simulink model "ICW_a1"  (Simulink 8.7)
settings: Solver=ode1  SolverMode=SingleTasking  StartTime=0.0  StopTime=500  FixedStep=0.001  RelTol=1e-3
(part 4 of 6)

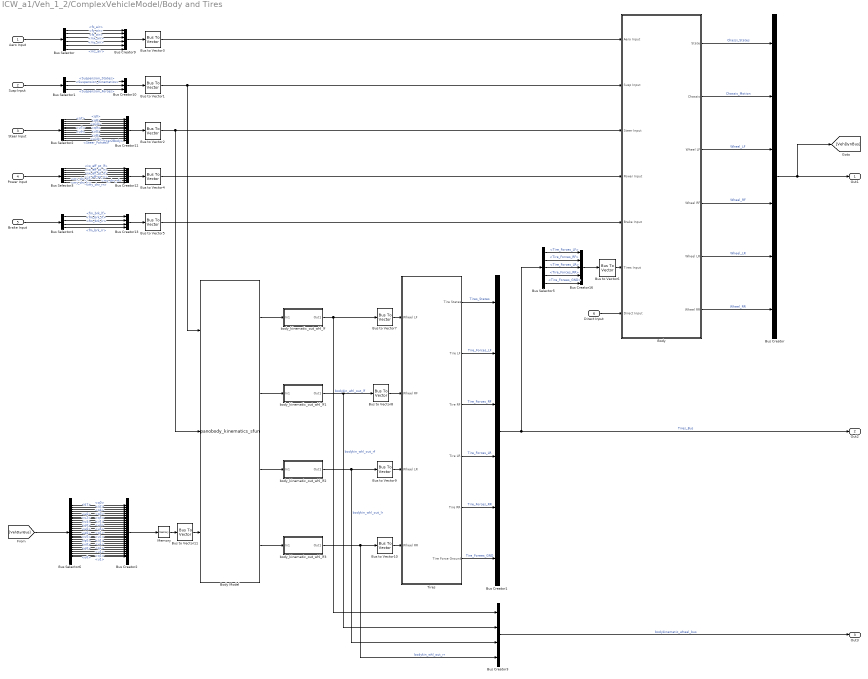
== system ICW_a1/Veh_1_2/ComplexVehicleModel/Body and Tires ==
  Aero Input : Inport
  Susp Input : Inport  Port=2
  Steer Input : Inport  Port=3
  Power Input : Inport  Port=4
  Brake Input : Inport  Port=5
  Direct Input : Inport  Port=6
  Body : Subsystem
  Body Model : S-Function  FunctionName=panobody_kinematics_sfun  Parameters='d84d7fde-53e6-4f2b-9c8e-847f55afb80f'  SFunctionDeploymentMode=off  EnableBusSupport=off
  Bus Creator : BusCreator  Inputs=6
  Bus Creator1 : BusCreator  Inputs=6
  Bus Creator10 : BusCreator  Inputs=3
  Bus Creator11 : BusCreator  Inputs=12
  Bus Creator12 : BusCreator  Inputs=8
  Bus Creator13 : BusCreator  Inputs=4
  Bus Creator16 : BusCreator  Inputs=5
  Bus Creator2 : BusCreator  Inputs=28
  Bus Creator3 : BusCreator  Inputs=4
  Bus Creator9 : BusCreator  Inputs=6
  Bus Selector : BusSelector  OutputSignals=Aerodynamics_Output.fx_air,Aerodynamics_Output.fy_air,Aerodynamics_Output.fz_air,Aerodynamics_Output.mx_air,Aerodynamics_Output.my_air,Aerodynamics_Output.mz_air
  Bus Selector1 : BusSelector  OutputSignals=Suspension_States,Suspension_Kinematics,Suspension_Forces
  Bus Selector2 : BusSelector  OutputSignals=Steer_States.q0,Steer_States.q7,Steer_States.q8,Steer_States.q9,Steer_States.q10,Steer_States.u0,Steer_States.u7,Steer_States.u8,Steer_States.u9,Steer_States.u10,Steer2Body,Steer_Forces
  Bus Selector3 : BusSelector  OutputSignals=Powertrain_Output.iw_eff_pt_lf,Powertrain_Output.iw_eff_pt_rf,Powertrain_Output.iw_eff_pt_lr,Powertrain_Output.iw_eff_pt_rr,Powertrain_Output.my_drv_lf,Powertrain_Output.my_drv_rf,Powertrain_Output.my_drv_lr,Powertrain_Output.my_drv_rr
  Bus Selector4 : BusSelector  OutputSignals=Brake_Output.fm_brk_lf,Brake_Output.fm_brk_rf,Brake_Output.fm_brk_lr,Brake_Output.fm_brk_rr
  Bus Selector5 : BusSelector  OutputSignals=Tire_Forces_LF,Tire_Forces_RF,Tire_Forces_LR,Tire_Forces_RR,Tire_Forees_GND
  Bus Selector6 : BusSelector  OutputSignals=Chassi_States.q0,Chassi_States.q1,Chassi_States.q2,Chassi_States.q3,Chassi_States.q4,Chassi_States.q5,Chassi_States.u0,Chassi_States.u1,Chassi_States.u2,Chassi_States.u3,Chassi_States.u4,Chassi_States.u5,Wheel_LF.q0,Wheel_LF.q1,Wheel_LF.u0,Wheel_LF.u1,Wheel_RF.q0,Wheel_RF.q1,Wheel_RF.u0,Wheel_RF.u1,Wheel_LR.q0,Wheel_LR.q1,Wheel_LR.u0,Wheel_LR.u1,Wheel_RR.q0,Wheel_RR.q1,Wheel_RR.u0,Wheel_RR.u1
  Bus to Vector{1..11} (11 alike) : BusToVector
  Memory : Memory
  Tires : Subsystem
  body_kinematic_out_whl_lf : Subsystem
  body_kinematic_out_whl_lf1 : Subsystem
  body_kinematic_out_whl_lf2 : Subsystem
  body_kinematic_out_whl_lf3 : Subsystem
  Out1 : Outport
  Out2 : Outport  Port=2
  Out3 : Outport  Port=3
  wires:
  Bus Selector5/5 -> Bus Creator16/5  "<Tire_Forees_GND>"
  Tires/6(Tire Force Ground) -> Bus Creator1/6  "Tire_Forees_GND"
  Aero Input/1 -> Bus Selector/1
  Susp Input/1 -> Bus Selector1/1
  Body/1(State) -> Bus Creator/1  "Chassi_States"
  Body/2(Chassis) -> Bus Creator/2  "Chassis_Motion"
  Body/3(Wheel LF) -> Bus Creator/3  "Wheel_LF"
  Body/4(Wheel RF) -> Bus Creator/4  "Wheel_RF"
  Body/5(Wheel LR) -> Bus Creator/5  "Wheel_LR"
  Body/6(Wheel RR) -> Bus Creator/6  "Wheel_RR"
  Bus Selector/1 -> Bus Creator9/1  "<fx_air>"
  Bus Selector/2 -> Bus Creator9/2  "<fy_air>"
  Bus Selector/3 -> Bus Creator9/3  "<fz_air>"
  Bus Selector/4 -> Bus Creator9/4  "<mx_air>"
  Bus Selector/5 -> Bus Creator9/5  "<my_air>"
  Bus Selector/6 -> Bus Creator9/6  "<mz_air>"
  Bus Selector1/1 -> Bus Creator10/1  "<Suspension_States>"
  Bus Selector1/2 -> Bus Creator10/2  "<Suspension_Kinematics>"
  Bus Selector3/1 -> Bus Creator12/1  "<iw_eff_pt_lf>"
  Bus Selector3/2 -> Bus Creator12/2  "<iw_eff_pt_rf>"
  Bus Selector3/3 -> Bus Creator12/3  "<iw_eff_pt_lr>"
  Bus Selector3/4 -> Bus Creator12/4  "<iw_eff_pt_rr>"
  Bus Selector4/1 -> Bus Creator13/1  "<fm_brk_lf>"
  Bus Selector4/2 -> Bus Creator13/2  "<fm_brk_rf>"
  Bus Selector4/3 -> Bus Creator13/3  "<fm_brk_lr>"
  Bus Selector4/4 -> Bus Creator13/4  "<fm_brk_rr>"
  Bus Selector5/1 -> Bus Creator16/1  "<Tire_Forces_LF>"
  Bus Selector5/2 -> Bus Creator16/2  "<Tire_Forces_RF>"
  Bus Selector5/3 -> Bus Creator16/3  "<Tire_Forces_LR>"
  Bus Selector5/4 -> Bus Creator16/4  "<Tire_Forces_RR>"
  Bus Creator16/1 -> Bus to Vector6/1
  Bus Selector2/1 -> Bus Creator11/1  "<q0>"
  Bus Selector2/2 -> Bus Creator11/2  "<q7>"
  Bus Selector2/3 -> Bus Creator11/3  "<q8>"
  Bus Selector2/4 -> Bus Creator11/4  "<q9>"
  Bus Selector2/5 -> Bus Creator11/5  "<q10>"
  Bus Selector2/6 -> Bus Creator11/6  "<u0>"
  Bus Selector2/7 -> Bus Creator11/7  "<u7>"
  Bus Selector2/8 -> Bus Creator11/8  "<u8>"
  Bus Selector2/9 -> Bus Creator11/9  "<u9>"
  Bus Selector2/10 -> Bus Creator11/10  "<u10>"
  Bus Selector2/11 -> Bus Creator11/11  "<Steer2Body>"
  Bus Selector2/12 -> Bus Creator11/12  "<Steer_Forces>"
  Bus Creator/1 -> Out1/1, [VehDynBus]
  Tires/1(Tire States) -> Bus Creator1/1  "Tires_States"
  Tires/2(Tire LF) -> Bus Creator1/2  "Tire_Forces_LF"
  Tires/3(Tire RF) -> Bus Creator1/3  "Tire_Forces_RF"
  Tires/4(Tire LR) -> Bus Creator1/4  "Tire_Forces_LR"
  Tires/5(Tire RR) -> Bus Creator1/5  "Tire_Forces_RR"
  Bus Creator1/1 -> Bus Selector5/1, Out2/1  "Tires_Bus"
  Power Input/1 -> Bus Selector3/1
  Direct Input/1 -> Body/7(Direct Input)
  Brake Input/1 -> Bus Selector4/1
  Body Model/1 -> body_kinematic_out_whl_lf/1(In1)
  Body Model/2 -> body_kinematic_out_whl_lf1/1(In1)
  Body Model/3 -> body_kinematic_out_whl_lf2/1(In1)
  Body Model/4 -> body_kinematic_out_whl_lf3/1(In1)
  Steer Input/1 -> Bus Selector2/1
  Bus Selector1/3 -> Bus Creator10/3  "<Suspension_Forces>"
  Bus Selector3/5 -> Bus Creator12/5  "<my_drv_lf>"
  Bus Selector3/6 -> Bus Creator12/6  "<my_drv_rf>"
  Bus Selector3/7 -> Bus Creator12/7  "<my_drv_lr>"
  Bus Selector3/8 -> Bus Creator12/8  "<my_drv_rr>"
  Bus Creator10/1 -> Bus to Vector1/1
  [VehDynBus] -> Bus Selector6/1
  Bus Selector6/1 -> Bus Creator2/1  "<q0>"
  Bus Selector6/2 -> Bus Creator2/2  "<q1>"
  Bus Selector6/3 -> Bus Creator2/3  "<q2>"
  Bus Selector6/4 -> Bus Creator2/4  "<q3>"
  Bus Selector6/5 -> Bus Creator2/5  "<q4>"
  Bus Selector6/6 -> Bus Creator2/6  "<q5>"
  Bus Selector6/7 -> Bus Creator2/7  "<u0>"
  Bus Selector6/8 -> Bus Creator2/8  "<u1>"
  Bus Selector6/9 -> Bus Creator2/9  "<u2>"
  Bus Selector6/10 -> Bus Creator2/10  "<u3>"
  Bus Selector6/11 -> Bus Creator2/11  "<u4>"
  Bus Selector6/12 -> Bus Creator2/12  "<u5>"
  Bus Selector6/13 -> Bus Creator2/13  "<q0>"
  Bus Selector6/14 -> Bus Creator2/14  "<q1>"
  Bus Selector6/15 -> Bus Creator2/15  "<u0>"
  Bus Selector6/16 -> Bus Creator2/16  "<u1>"
  Bus Selector6/17 -> Bus Creator2/17  "<q0>"
  Bus Selector6/18 -> Bus Creator2/18  "<q1>"
  Bus Selector6/19 -> Bus Creator2/19  "<u0>"
  Bus Selector6/20 -> Bus Creator2/20  "<u1>"
  Bus Selector6/21 -> Bus Creator2/21  "<q0>"
  Bus Selector6/22 -> Bus Creator2/22  "<q1>"
  Bus Selector6/23 -> Bus Creator2/23  "<u0>"
  Bus Selector6/24 -> Bus Creator2/24  "<u1>"
  Bus Selector6/25 -> Bus Creator2/25  "<q0>"
  Bus Selector6/26 -> Bus Creator2/26  "<q1>"
  Bus Selector6/27 -> Bus Creator2/27  "<u0>"
  Bus Selector6/28 -> Bus Creator2/28  "<u1>"
  Bus Creator2/1 -> Memory/1
  Memory/1 -> Bus to Vector11/1
  Bus Creator11/1 -> Bus to Vector2/1
  Bus Creator9/1 -> Bus to Vector3/1
  Bus Creator12/1 -> Bus to Vector4/1
  Bus Creator13/1 -> Bus to Vector5/1
  body_kinematic_out_whl_lf/1(Out1) -> Bus to Vector7/1, Bus Creator3/1  "bodykin_whl_out_lf"
  body_kinematic_out_whl_lf1/1(Out1) -> Bus to Vector8/1, Bus Creator3/2  "bodykin_whl_out_rf"
  body_kinematic_out_whl_lf2/1(Out1) -> Bus to Vector9/1, Bus Creator3/3  "bodykin_whl_out_lr"
  body_kinematic_out_whl_lf3/1(Out1) -> Bus to Vector10/1, Bus Creator3/4  "bodykin_whl_out_rr"
  Bus Creator3/1 -> Out3/1  "bodykinematic_wheel_bus"
  Bus to Vector3/1 -> Body/1(Aero Input)
  Bus to Vector1/1 -> Body/2(Susp Input), Body Model/1
  Bus to Vector2/1 -> Body/3(Steer Input), Body Model/2
  Bus to Vector4/1 -> Body/4(Power Input)
  Bus to Vector5/1 -> Body/5(Brake Input)
  Bus to Vector6/1 -> Body/6(Tires Input)
  Bus to Vector7/1 -> Tires/1(Wheel LF)
  Bus to Vector8/1 -> Tires/2(Wheel RF)
  Bus to Vector9/1 -> Tires/3(Wheel LR)
  Bus to Vector10/1 -> Tires/4(Wheel RR)
  Bus to Vector11/1 -> Body Model/3

== system ICW_a1/Veh_1_2/ComplexVehicleModel/Brake ==
  Body Input : Inport
  Driver Input : Inport  Port=2
  Inertia Wheel : Inport  Port=3
  Fz Wheel : Inport  Port=4
  Direct Input : Inport  Port=5
  Brake Model : S-Function  FunctionName=panoBrake_sfun  Parameters='d84d7fde-53e6-4f2b-9c8e-847f55afb80f'  SFunctionDeploymentMode=off  EnableBusSupport=off
  Brake States : Subsystem
  Memory : Memory
  SteerStates1 : Subsystem
  BrakeStates : Outport
  BrakeOutput : Outport  Port=2
  wires:
  Direct Input/1 -> Brake Model/5
  Brake Model/1 -> Brake States/1(In1)
  Brake Model/2 -> SteerStates1/1(In1)
  Body Input/1 -> Memory/1
  Driver Input/1 -> Brake Model/2
  Inertia Wheel/1 -> Brake Model/3
  Fz Wheel/1 -> Brake Model/4
  Brake States/1(Out1) -> BrakeStates/1
  SteerStates1/1(Out1) -> BrakeOutput/1
  Memory/1 -> Brake Model/1

== system ICW_a1/Veh_1_2/ComplexVehicleModel/Powertrain ==
  Body Input : Inport
  Throttle : Inport  Port=2
  TransMode : Inport  Port=3
  Gear : Inport  Port=4
  BrakeSignal : Inport  Port=5
  Memory : Memory
  Powertrain Model : S-Function  FunctionName=panoPowertrain_sfun  Parameters='d84d7fde-53e6-4f2b-9c8e-847f55afb80f'  SFunctionDeploymentMode=off  EnableBusSupport=off
  PowertrainOut : Subsystem
  PowertrainStates : Subsystem
  Powertrain States : Outport
  Powertrain Output : Outport  Port=2
  wires:
  BrakeSignal/1 -> Powertrain Model/5
  Gear/1 -> Powertrain Model/4
  TransMode/1 -> Powertrain Model/3
  Throttle/1 -> Powertrain Model/2
  Powertrain Model/1 -> PowertrainStates/1(In1)
  PowertrainStates/1(Out1) -> Powertrain States/1
  PowertrainOut/1(Out1) -> Powertrain Output/1
  Powertrain Model/2 -> PowertrainOut/1(In1)
  Memory/1 -> Powertrain Model/1
  Body Input/1 -> Memory/1

== system ICW_a1/Veh_1_2/ComplexVehicleModel/Steer ==
  Body Input : Inport
  Steer Angle : Inport  Port=2
  Suspension Input : Inport  Port=3
  Tire Input : Inport  Port=4
  Direct Steer : Inport  Port=5
  Memory : Memory
  Memory1 : Memory
  SteerForces : Subsystem
  SteerKinemateics : Subsystem
  SteerStates : Subsystem
  SteerToBody : Subsystem
  Steering Model : S-Function  FunctionName=panoSteer_sfun  Parameters='d84d7fde-53e6-4f2b-9c8e-847f55afb80f'  SFunctionDeploymentMode=off  EnableBusSupport=off
  Steer States : Outport
  Steer Kinematiocs : Outport  Port=2
  Steer2Body : Outport  Port=3
  Steer Forces : Outport  Port=4
  wires:
  Direct Steer/1 -> Steering Model/5
  Body Input/1 -> Memory/1
  Suspension Input/1 -> Steering Model/3
  Tire Input/1 -> Memory1/1
  Steer Angle/1 -> Steering Model/2
  Steering Model/1 -> SteerStates/1(In1)
  SteerStates/1(Out1) -> Steer States/1  "Steer_States"
  SteerKinemateics/1(Out1) -> Steer Kinematiocs/1  "Steer_Kinematics"
  SteerToBody/1(Out1) -> Steer2Body/1  "SteertoBody"
  SteerForces/1(Out1) -> Steer Forces/1  "Steer_Forces"
  Steering Model/2 -> SteerKinemateics/1(In1)
  Steering Model/3 -> SteerToBody/1(In1)
  Steering Model/4 -> SteerForces/1(In1)
  Memory/1 -> Steering Model/1
  Memory1/1 -> Steering Model/4

== system ICW_a1/Veh_1_2/ComplexVehicleModel/Suspensions ==
  Body Input : Inport
  WheelLF Input : Inport  Port=2
  WheelRF Input : Inport  Port=3
  WheelLR Input : Inport  Port=4
  WheelRR Input : Inport  Port=5
  Memory{,1..4} (5 alike) : Memory
  SupensionsStates : Subsystem
  Suspension Model : S-Function  FunctionName=panoSuspension_sfun  Parameters='d84d7fde-53e6-4f2b-9c8e-847f55afb80f'  SFunctionDeploymentMode=off  EnableBusSupport=off
  SuspensionForces : Subsystem
  SuspensionKinematics : Subsystem
  SuspensionSteer : Subsystem
  Suspensions States : Outport
  Suspension Kinematics : Outport  Port=2
  Suspension Forces : Outport  Port=3
  Suspension Steer : Outport  Port=4
  wires:
  Body Input/1 -> Memory/1
  WheelLF Input/1 -> Memory1/1
  WheelRF Input/1 -> Memory2/1
  WheelLR Input/1 -> Memory3/1
  WheelRR Input/1 -> Memory4/1
  Suspension Model/1 -> SupensionsStates/1(In1)
  SupensionsStates/1(Out1) -> Suspensions States/1  "Supension_States"
  SuspensionKinematics/1(Out1) -> Suspension Kinematics/1  "Suspension_Kinematics"
  SuspensionForces/1(Out1) -> Suspension Forces/1  "Suspension_Forces"
  SuspensionSteer/1(Out1) -> Suspension Steer/1  "Suspension_Steer"
  Suspension Model/2 -> SuspensionKinematics/1(In1)
  Suspension Model/3 -> SuspensionForces/1(In1)
  Suspension Model/4 -> SuspensionSteer/1(In1)
  Memory/1 -> Suspension Model/1
  Memory1/1 -> Suspension Model/2
  Memory2/1 -> Suspension Model/3
  Memory3/1 -> Suspension Model/4
  Memory4/1 -> Suspension Model/5

== system ICW_a1/Veh_1_2/DriverModel/Driver ==
  Body Input : Inport
  Steer Input : Inport  Port=2
  Engine Input : Inport  Port=3
  Brake Input : Inport  Port=4
  Bus to Vector1 : BusToVector
  Bus to Vector2 : BusToVector
  Bus to Vector3 : BusToVector
  Driver Model : S-Function  FunctionName=panoDriver_sfun  Parameters='d84d7fde-53e6-4f2b-9c8e-847f55afb80f'  SFunctionDeploymentMode=off  EnableBusSupport=off
  Driver2Brake : Subsystem
  Driver2Powertrain : Subsystem
  Driver2Steer : Subsystem
  DriverStates : Subsystem
  Memory{,1..3} (4 alike) : Memory
  Driver_States : Outport
  Driver_Steer : Outport  Port=2
  Driver_Powertrain : Outport  Port=3
  Driver_Brake : Outport  Port=4
  wires:
  Memory3/1 -> Driver Model/4
  Memory2/1 -> Bus to Vector3/1
  Memory1/1 -> Bus to Vector1/1
  Memory/1 -> Bus to Vector2/1
  Body Input/1 -> Memory/1
  Steer Input/1 -> Memory1/1
  Driver2Powertrain/1(Out1) -> Driver_Powertrain/1
  Driver2Brake/1(Out1) -> Driver_Brake/1
  Driver Model/4 -> Driver2Brake/1(In1)
  Driver Model/3 -> Driver2Powertrain/1(In1)
  Driver2Steer/1(Out1) -> Driver_Steer/1
  Driver Model/2 -> Driver2Steer/1(In1)
  DriverStates/1(Out1) -> Driver_States/1
  Driver Model/1 -> DriverStates/1(In1)
  Engine Input/1 -> Memory2/1
  Brake Input/1 -> Memory3/1
  Bus to Vector2/1 -> Driver Model/1
  Bus to Vector1/1 -> Driver Model/2
  Bus to Vector3/1 -> Driver Model/3

== system ICW_a1/Veh_1/ComplexVehicleModel/Aerodynamics/Chassis States ==
  In1 : Inport
  Bus Creator : BusCreator  Inputs=12
  Demux : Demux  Outputs=12
  Out1 : Outport
  wires:
  In1/1 -> Demux/1
  Demux/1 -> Bus Creator/1  "beta_air"
  Demux/2 -> Bus Creator/2  "pitch_air"
  Demux/3 -> Bus Creator/3  "yawwind_air"
  Demux/4 -> Bus Creator/4  "v_air"
  Demux/5 -> Bus Creator/5  "vwind_air"
  Demux/6 -> Bus Creator/6  "z_air"
  Demux/7 -> Bus Creator/7  "fx_air"
  Demux/8 -> Bus Creator/8  "fy_air"
  Demux/9 -> Bus Creator/9  "fz_air"
  Demux/10 -> Bus Creator/10  "mx_air"
  Demux/11 -> Bus Creator/11  "my_air"
  Demux/12 -> Bus Creator/12  "mz_air"
  Bus Creator/1 -> Out1/1  "Aerodynamics_States"

== system ICW_a1/Veh_1/ComplexVehicleModel/Body and Tires/Body ==
  Aero Input : Inport
  Susp Input : Inport  Port=2
  Steer Input : Inport  Port=3
  Power Input : Inport  Port=4
  Brake Input : Inport  Port=5
  Tires Input : Inport  Port=6
  Direct Input : Inport  Port=7
  Body Model : S-Function  FunctionName=panoBody_sfun  Parameters='7a840300-6a2b-4f34-9d95-831f7d6ae28e'  SFunctionDeploymentMode=off  EnableBusSupport=off
  Chassis Motion : Subsystem
  Chassis States : Subsystem
  Wheel 1 : Subsystem
  Wheel 2 : Subsystem
  Wheel 3 : Subsystem
  Wheel 4 : Subsystem
  State : Outport
  Chassis : Outport  Port=2
  Wheel LF : Outport  Port=3
  Wheel RF : Outport  Port=4
  Wheel LR : Outport  Port=5
  Wheel RR : Outport  Port=6
  wires:
  Direct Input/1 -> Body Model/7
  Body Model/2 -> Chassis Motion/1(In1)
  Chassis Motion/1(Out1) -> Chassis/1  "Chassis_Motion"
  Body Model/1 -> Chassis States/1(In1)
  Chassis States/1(Out1) -> State/1  "Chassis_States"
  Body Model/3 -> Wheel 1/1(In1)
  Wheel 1/1(Out1) -> Wheel LF/1  "Wheel_LF"
  Body Model/4 -> Wheel 2/1(In1)
  Body Model/5 -> Wheel 3/1(In1)
  Body Model/6 -> Wheel 4/1(In1)
  Wheel 3/1(Out1) -> Wheel LR/1  "Wheel_LR"
  Wheel 4/1(Out1) -> Wheel RR/1  "Wheel_RR"
  Wheel 2/1(Out1) -> Wheel RF/1  "Wheel_RF"
  Tires Input/1 -> Body Model/6
  Power Input/1 -> Body Model/4
  Brake Input/1 -> Body Model/5
  Steer Input/1 -> Body Model/3
  Susp Input/1 -> Body Model/2
  Aero Input/1 -> Body Model/1

== system ICW_a1/Veh_1/ComplexVehicleModel/Body and Tires/Tires ==
  Wheel LF : Inport
  Wheel RF : Inport  Port=2
  Wheel LR : Inport  Port=3
  Wheel RR : Inport  Port=4
  Tires Force  2 : Subsystem
  "Tires Force 1 " : Subsystem
  Tires Force 3 : Subsystem
  Tires Force 4 : Subsystem
  Tires Force Ground : Subsystem
  Tires Model : S-Function  FunctionName=panoTire_sfun  Parameters='7a840300-6a2b-4f34-9d95-831f7d6ae28e'  SFunctionDeploymentMode=off  EnableBusSupport=off
  TiresStates : Subsystem
  Tire States : Outport
  Tire LF : Outport  Port=2
  Tire RF : Outport  Port=3
  Tire LR : Outport  Port=4
  Tire RR : Outport  Port=5
  Tire Force Ground : Outport  Port=6
  wires:
  Tires Model/6 -> Tires Force Ground/1(In1)
  Tires Force Ground/1(Out1) -> Tire Force Ground/1  "Tire_Forces_GND"
  Wheel LF/1 -> Tires Model/1
  Wheel RF/1 -> Tires Model/2
  Wheel LR/1 -> Tires Model/3
  Wheel RR/1 -> Tires Model/4
  Tires Model/1 -> TiresStates/1(In1)
  TiresStates/1(Out1) -> Tire States/1  "Tires_States"
  Tires Model/2 -> "Tires Force 1 "/1(In1)
  "Tires Force 1 "/1(Out1) -> Tire LF/1  "Tire_Forces_LF"
  Tires Model/5 -> Tires Force 4/1(In1)
  Tires Model/4 -> Tires Force 3/1(In1)
  Tires Model/3 -> Tires Force  2/1(In1)
  Tires Force 3/1(Out1) -> Tire LR/1  "Tire_Forces_LR"
  Tires Force 4/1(Out1) -> Tire RR/1  "Tire_Forces_RR"
  Tires Force  2/1(Out1) -> Tire RF/1  "Tire_Forces_RF"

== system ICW_a1/Veh_1/ComplexVehicleModel/Body and Tires/body_kinematic_out_whl_lf ==
  In1 : Inport
  Bus Creator : BusCreator  Inputs=18
  Demux : Demux  Outputs=18
  Out1 : Outport
  wires:
  In1/1 -> Demux/1
  Demux/1 -> Bus Creator/1  "rot_whl"
  Demux/2 -> Bus Creator/2  "w_whl"
  Demux/3 -> Bus Creator/3  "z_whl_whl"
  Demux/4 -> Bus Creator/4  "yaw_whl"
  Demux/5 -> Bus Creator/5  "pitch_whl"
  Demux/6 -> Bus Creator/6  "roll_whl"
  Demux/7 -> Bus Creator/7  "vwx_whl"
  Demux/8 -> Bus Creator/8  "vwy_whl"
  Demux/9 -> Bus Creator/9  "vwz_whl"
  Demux/10 -> Bus Creator/10  "avwx_whl"
  Demux/11 -> Bus Creator/11  "avwy_whl"
  Demux/12 -> Bus Creator/12  "avwz_whl"
  Demux/13 -> Bus Creator/13  "dzdx_whl"
  Demux/14 -> Bus Creator/14  "dzdy_whl"
  Demux/15 -> Bus Creator/15  "xgnd_whl"
  Demux/16 -> Bus Creator/16  "ygnd_whl"
  Demux/17 -> Bus Creator/17  "zgnd_whl"
  Demux/18 -> Bus Creator/18  "mux_whl"
  Bus Creator/1 -> Out1/1  "bodykin_whl_out"

== system ICW_a1/Veh_1/ComplexVehicleModel/Body and Tires/body_kinematic_out_whl_lf1 ==
  In1 : Inport
  Bus Creator : BusCreator  Inputs=18
  Demux : Demux  Outputs=18
  Out1 : Outport
  wires:
  Bus Creator/1 -> Out1/1  "bodykin_whl_out"
  Demux/18 -> Bus Creator/18  "mux_whl"
  Demux/17 -> Bus Creator/17  "zgnd_whl"
  Demux/16 -> Bus Creator/16  "ygnd_whl"
  Demux/15 -> Bus Creator/15  "xgnd_whl"
  Demux/14 -> Bus Creator/14  "dzdy_whl"
  Demux/13 -> Bus Creator/13  "dzdx_whl"
  Demux/12 -> Bus Creator/12  "avwz_whl"
  Demux/11 -> Bus Creator/11  "avwy_whl"
  Demux/10 -> Bus Creator/10  "avwx_whl"
  Demux/9 -> Bus Creator/9  "vwz_whl"
  Demux/8 -> Bus Creator/8  "vwy_whl"
  Demux/7 -> Bus Creator/7  "vwx_whl"
  Demux/6 -> Bus Creator/6  "roll_whl"
  Demux/5 -> Bus Creator/5  "pitch_whl"
  Demux/4 -> Bus Creator/4  "yaw_whl"
  Demux/3 -> Bus Creator/3  "z_whl_whl"
  Demux/2 -> Bus Creator/2  "w_whl"
  Demux/1 -> Bus Creator/1  "rot_whl"
  In1/1 -> Demux/1

== system ICW_a1/Veh_1/ComplexVehicleModel/Body and Tires/body_kinematic_out_whl_lf2 ==
  In1 : Inport
  Bus Creator : BusCreator  Inputs=18
  Demux : Demux  Outputs=18
  Out1 : Outport
  wires:
  In1/1 -> Demux/1
  Demux/1 -> Bus Creator/1  "rot_whl"
  Demux/2 -> Bus Creator/2  "w_whl"
  Demux/3 -> Bus Creator/3  "z_whl_whl"
  Demux/4 -> Bus Creator/4  "yaw_whl"
  Demux/5 -> Bus Creator/5  "pitch_whl"
  Demux/6 -> Bus Creator/6  "roll_whl"
  Demux/7 -> Bus Creator/7  "vwx_whl"
  Demux/8 -> Bus Creator/8  "vwy_whl"
  Demux/9 -> Bus Creator/9  "vwz_whl"
  Demux/10 -> Bus Creator/10  "avwx_whl"
  Demux/11 -> Bus Creator/11  "avwy_whl"
  Demux/12 -> Bus Creator/12  "avwz_whl"
  Demux/13 -> Bus Creator/13  "dzdx_whl"
  Demux/14 -> Bus Creator/14  "dzdy_whl"
  Demux/15 -> Bus Creator/15  "xgnd_whl"
  Demux/16 -> Bus Creator/16  "ygnd_whl"
  Demux/17 -> Bus Creator/17  "zgnd_whl"
  Demux/18 -> Bus Creator/18  "mux_whl"
  Bus Creator/1 -> Out1/1  "bodykin_whl_out"

== system ICW_a1/Veh_1/ComplexVehicleModel/Body and Tires/body_kinematic_out_whl_lf3 ==
  In1 : Inport
  Bus Creator : BusCreator  Inputs=18
  Demux : Demux  Outputs=18
  Out1 : Outport
  wires:
  Bus Creator/1 -> Out1/1  "bodykin_whl_out"
  Demux/18 -> Bus Creator/18  "mux_whl"
  Demux/17 -> Bus Creator/17  "zgnd_whl"
  Demux/16 -> Bus Creator/16  "ygnd_whl"
  Demux/15 -> Bus Creator/15  "xgnd_whl"
  Demux/14 -> Bus Creator/14  "dzdy_whl"
  Demux/13 -> Bus Creator/13  "dzdx_whl"
  Demux/12 -> Bus Creator/12  "avwz_whl"
  Demux/11 -> Bus Creator/11  "avwy_whl"
  Demux/10 -> Bus Creator/10  "avwx_whl"
  Demux/9 -> Bus Creator/9  "vwz_whl"
  Demux/8 -> Bus Creator/8  "vwy_whl"
  Demux/7 -> Bus Creator/7  "vwx_whl"
  Demux/6 -> Bus Creator/6  "roll_whl"
  Demux/5 -> Bus Creator/5  "pitch_whl"
  Demux/4 -> Bus Creator/4  "yaw_whl"
  Demux/3 -> Bus Creator/3  "z_whl_whl"
  Demux/2 -> Bus Creator/2  "w_whl"
  Demux/1 -> Bus Creator/1  "rot_whl"
  In1/1 -> Demux/1

== system ICW_a1/Veh_1/ComplexVehicleModel/Brake/Brake States ==
  In1 : Inport
  Bus Creator : BusCreator  Inputs=26
  Demux : Demux  Outputs=26
  Out1 : Outport
  wires:
  In1/1 -> Demux/1
  Demux/1 -> Bus Creator/1  "q0"
  Demux/2 -> Bus Creator/2  "q1"
  Demux/3 -> Bus Creator/3  "q2"
  Demux/4 -> Bus Creator/4  "q3"
  Demux/5 -> Bus Creator/5  "q4"
  Demux/6 -> Bus Creator/6  "q5"
  Demux/7 -> Bus Creator/7  "q6"
  Demux/8 -> Bus Creator/8  "q7"
  Demux/9 -> Bus Creator/9  "q8"
  Demux/10 -> Bus Creator/10  "q9"
  Demux/11 -> Bus Creator/11  "q10"
  Demux/12 -> Bus Creator/12  "q11"
  Demux/13 -> Bus Creator/13  "q12"
  Demux/14 -> Bus Creator/14  "u0"
  Demux/15 -> Bus Creator/15  "u1"
  Demux/16 -> Bus Creator/16  "u2"
  Bus Creator/1 -> Out1/1  "BrakeStates"
  Demux/17 -> Bus Creator/17  "u3"
  Demux/18 -> Bus Creator/18  "u4"
  Demux/19 -> Bus Creator/19  "u5"
  Demux/20 -> Bus Creator/20  "u6"
  Demux/21 -> Bus Creator/21  "u7"
  Demux/22 -> Bus Creator/22  "u8"
  Demux/23 -> Bus Creator/23  "u9"
  Demux/24 -> Bus Creator/24  "u10"
  Demux/25 -> Bus Creator/25  "u11"
  Demux/26 -> Bus Creator/26  "u12"

== system ICW_a1/Veh_1/ComplexVehicleModel/Brake/SteerStates1 ==
  In1 : Inport
  Bus Creator : BusCreator  Inputs=22
  Demux : Demux  Outputs=22
  Out1 : Outport
  wires:
  Demux/22 -> Bus Creator/22  "turn_off"
  Demux/21 -> Bus Creator/21  "brake"
  Demux/20 -> Bus Creator/20  "trot_brk_rr"
  Demux/19 -> Bus Creator/19  "trot_brk_lr"
  Demux/18 -> Bus Creator/18  "trot_brk_rf"
  Demux/17 -> Bus Creator/17  "trot_brk_lf"
  Bus Creator/1 -> Out1/1  "BrakeOutput"
  Demux/16 -> Bus Creator/16  "mu_us_brk_rr"
  Demux/15 -> Bus Creator/15  "mu_us_brk_lr"
  Demux/14 -> Bus Creator/14  "mu_us_brk_rf"
  Demux/13 -> Bus Creator/13  "mu_us_brk_lf"
  Demux/12 -> Bus Creator/12  "fm_brk_rr"
  Demux/11 -> Bus Creator/11  "fm_brk_lr"
  Demux/10 -> Bus Creator/10  "fm_brk_rf"
  Demux/9 -> Bus Creator/9  "fm_brk_lf"
  Demux/8 -> Bus Creator/8  "pbkch_brk_rr"
  Demux/7 -> Bus Creator/7  "pbkch_brk_lr"
  Demux/6 -> Bus Creator/6  "pbkch_brk_rf"
  Demux/5 -> Bus Creator/5  "pbkch_brk_lf"
  Demux/4 -> Bus Creator/4  "fbk_out_brk"
  Demux/3 -> Bus Creator/3  "fbk_in_brk"
  Demux/2 -> Bus Creator/2  "fbk_pedal"
  Demux/1 -> Bus Creator/1  "pbk_con_brk"
  In1/1 -> Demux/1

== system ICW_a1/Veh_1/ComplexVehicleModel/Powertrain/PowertrainOut ==
  In1 : Inport
  Bus Creator : BusCreator  Inputs=36
  Demux : Demux  Outputs=36
  Out1 : Outport
  wires:
  Bus Creator/1 -> Out1/1  "PowertrainOut"
  In1/1 -> Demux/1
  Demux/1 -> Bus Creator/1  "aa_eng"
  Demux/2 -> Bus Creator/2  "av_eng"
  Demux/3 -> Bus Creator/3  "av_eng_update"
  Demux/4 -> Bus Creator/4  "av_tc"
  Demux/5 -> Bus Creator/5  "fuel"
  Demux/6 -> Bus Creator/6  "iw_eff_pt_lf"
  Demux/7 -> Bus Creator/7  "iw_eff_pt_rf"
  Demux/8 -> Bus Creator/8  "iw_eff_pt_lr"
  Demux/9 -> Bus Creator/9  "iw_eff_pt_rr"
  Demux/10 -> Bus Creator/10  "my_drv_lf"
  Demux/11 -> Bus Creator/11  "my_drv_rf"
  Demux/12 -> Bus Creator/12  "my_drv_lr"
  Demux/13 -> Bus Creator/13  "my_drv_rr"
  Demux/14 -> Bus Creator/14  "pt_thr_eng"
  Demux/15 -> Bus Creator/15  "pt_throttle"
  Demux/16 -> Bus Creator/16  "pt_modetran"
  Demux/17 -> Bus Creator/17  "pt_rottrans"
  Demux/18 -> Bus Creator/18  "pt_m_engout"
  Demux/19 -> Bus Creator/19  "pt_m_eng_in"
  Demux/20 -> Bus Creator/20  "pt_gearauto"
  Demux/21 -> Bus Creator/21  "pt_gear_status"
  Demux/22 -> Bus Creator/22  "pt_gear_man"
  Demux/23 -> Bus Creator/23  "rot_eng_update"
  Demux/24 -> Bus Creator/24  "rot_tc"
  Demux/25 -> Bus Creator/25  "pt_av_trans"
  Demux/26 -> Bus Creator/26  "pt_m_tc"
  Demux/27 -> Bus Creator/27  "pt_m_trans"
  Demux/28 -> Bus Creator/28  "pt_pwrengin"
  Demux/29 -> Bus Creator/29  "pt_pwrengo"
  Demux/30 -> Bus Creator/30  "pt_pwrtrans"
  Demux/31 -> Bus Creator/31  "pt_pwrwheel"
  Demux/32 -> Bus Creator/32  "pt_pwr_tc"
  Demux/33 -> Bus Creator/33  "pt_clutch"
  Demux/34 -> Bus Creator/34  "pt_k_tc"
  Demux/35 -> Bus Creator/35  "pt_r_av_tc"
  Demux/36 -> Bus Creator/36  "pt_r_m_tc"

== system ICW_a1/Veh_1/ComplexVehicleModel/Powertrain/PowertrainStates ==
  In1 : Inport
  Bus Creator : BusCreator  Inputs=38
  Demux : Demux  Outputs=38
  Out1 : Outport
  wires:
  In1/1 -> Demux/1
  Bus Creator/1 -> Out1/1  "PowertrainStates"
  Demux/1 -> Bus Creator/1  "q0"
  Demux/2 -> Bus Creator/2  "q1"
  Demux/3 -> Bus Creator/3  "q2"
  Demux/4 -> Bus Creator/4  "q3"
  Demux/5 -> Bus Creator/5  "q4"
  Demux/6 -> Bus Creator/6  "q5"
  Demux/7 -> Bus Creator/7  "q6"
  Demux/8 -> Bus Creator/8  "q7"
  Demux/9 -> Bus Creator/9  "q8"
  Demux/10 -> Bus Creator/10  "q9"
  Demux/11 -> Bus Creator/11  "q10"
  Demux/12 -> Bus Creator/12  "q11"
  Demux/13 -> Bus Creator/13  "q12"
  Demux/14 -> Bus Creator/14  "q13"
  Demux/15 -> Bus Creator/15  "q14"
  Demux/16 -> Bus Creator/16  "q15"
  Demux/17 -> Bus Creator/17  "q16"
  Demux/18 -> Bus Creator/18  "q17"
  Demux/19 -> Bus Creator/19  "q18"
  Demux/20 -> Bus Creator/20  "u0"
  Demux/21 -> Bus Creator/21  "u1"
  Demux/22 -> Bus Creator/22  "u2"
  Demux/23 -> Bus Creator/23  "u3"
  Demux/24 -> Bus Creator/24  "u4"
  Demux/25 -> Bus Creator/25  "u5"
  Demux/26 -> Bus Creator/26  "u6"
  Demux/27 -> Bus Creator/27  "u7"
  Demux/28 -> Bus Creator/28  "u8"
  Demux/29 -> Bus Creator/29  "u9"
  Demux/30 -> Bus Creator/30  "u10"
  Demux/31 -> Bus Creator/31  "u11"
  Demux/32 -> Bus Creator/32  "u12"
  Demux/33 -> Bus Creator/33  "u13"
  Demux/34 -> Bus Creator/34  "u14"
  Demux/35 -> Bus Creator/35  "u15"
  Demux/36 -> Bus Creator/36  "u16"
  Demux/37 -> Bus Creator/37  "u17"
  Demux/38 -> Bus Creator/38  "u18"

== system ICW_a1/Veh_1/ComplexVehicleModel/Steer/SteerForces ==
  In1 : Inport
  Bus Creator : BusCreator  Inputs=32
  Demux : Demux  Outputs=32
  Out1 : Outport
  wires:
  Bus Creator/1 -> Out1/1  "Steer_Forces"
  Demux/26 -> Bus Creator/26  "steer_f_hys_2"
  Demux/25 -> Bus Creator/25  "steer_f_hys_1"
  Demux/24 -> Bus Creator/24  "steer_mkp_in_4"
  Demux/23 -> Bus Creator/23  "steer_mkp_in_3"
  Demux/22 -> Bus Creator/22  "steer_mkp_in_2"
  Demux/21 -> Bus Creator/21  "steer_mkp_in_1"
  Demux/20 -> Bus Creator/20  "steer_gear_dam_f_2"
  Demux/19 -> Bus Creator/19  "steer_boost_f_2"
  Demux/18 -> Bus Creator/18  "steer_gear_dam_t_2"
  Demux/17 -> Bus Creator/17  "steer_boost_t_2"
  Demux/16 -> Bus Creator/16  "steer_gear_dam_f_1"
  Demux/15 -> Bus Creator/15  "steer_boost_f_1"
  Demux/14 -> Bus Creator/14  "steer_gear_dam_t_1"
  Demux/13 -> Bus Creator/13  "steer_boost_t_1"
  Demux/12 -> Bus Creator/12  "steer_col_fric_t3"
  Demux/11 -> Bus Creator/11  "steer_col_dam_t3"
  Demux/10 -> Bus Creator/10  "steer_col_fric_t2"
  Demux/9 -> Bus Creator/9  "steer_col_dam_t2"
  Demux/8 -> Bus Creator/8  "steer_t_in1"
  Demux/7 -> Bus Creator/7  "steer_tbar_t1"
  Demux/6 -> Bus Creator/6  "steer_col_fric_t1"
  Demux/5 -> Bus Creator/5  "steer_col_dam_t1"
  Demux/4 -> Bus Creator/4  "steer_tbar_t"
  Demux/3 -> Bus Creator/3  "steer_col_fric_t"
  Demux/2 -> Bus Creator/2  "steer_col_dam_t"
  Demux/1 -> Bus Creator/1  "steer_t_in"
  In1/1 -> Demux/1
  Demux/27 -> Bus Creator/27  "steer_f_hys_3"
  Demux/28 -> Bus Creator/28  "steer_f_hys_4"
  Demux/29 -> Bus Creator/29  "m_kp_str_1"
  Demux/30 -> Bus Creator/30  "m_kp_str_2"
  Demux/31 -> Bus Creator/31  "m_kp_str_3"
  Demux/32 -> Bus Creator/32  "m_kp_str_4"

== system ICW_a1/Veh_1/ComplexVehicleModel/Steer/SteerKinemateics ==
  In1 : Inport
  Bus Creator : BusCreator  Inputs=9
  Demux : Demux  Outputs=[4 1 1 1 1 4 4 4 2]
  Out1 : Outport
  wires:
  Bus Creator/1 -> Out1/1  "Steer_Kinematics"
  Demux/8 -> Bus Creator/8  "k_str"
  Demux/7 -> Bus Creator/7  "c_str"
  Demux/6 -> Bus Creator/6  "steer_str"
  Demux/5 -> Bus Creator/5  "str_sus_r"
  Demux/4 -> Bus Creator/4  "str_sus_f"
  Demux/3 -> Bus Creator/3  "strav_sw"
  Demux/2 -> Bus Creator/2  "drstr"
  Demux/1 -> Bus Creator/1  "str_whl_opt"
  In1/1 -> Demux/1
  Demux/9 -> Bus Creator/9  "strswr"

== system ICW_a1/Veh_1/ComplexVehicleModel/Steer/SteerStates ==
  In1 : Inport
  Bus Creator : BusCreator  Inputs=26
  Demux : Demux  Outputs=26
  Out1 : Outport
  wires:
  In1/1 -> Demux/1
  Demux/1 -> Bus Creator/1  "q0"
  Demux/2 -> Bus Creator/2  "q1"
  Demux/3 -> Bus Creator/3  "q2"
  Demux/4 -> Bus Creator/4  "q3"
  Demux/5 -> Bus Creator/5  "q4"
  Demux/6 -> Bus Creator/6  "q5"
  Demux/7 -> Bus Creator/7  "q6"
  Demux/8 -> Bus Creator/8  "q7"
  Demux/9 -> Bus Creator/9  "q8"
  Demux/10 -> Bus Creator/10  "q9"
  Demux/11 -> Bus Creator/11  "q10"
  Demux/12 -> Bus Creator/12  "q11"
  Demux/13 -> Bus Creator/13  "q12"
  Demux/14 -> Bus Creator/14  "u0"
  Demux/15 -> Bus Creator/15  "u1"
  Demux/16 -> Bus Creator/16  "u2"
  Bus Creator/1 -> Out1/1  "SteerStates"
  Demux/17 -> Bus Creator/17  "u3"
  Demux/18 -> Bus Creator/18  "u4"
  Demux/19 -> Bus Creator/19  "u5"
  Demux/20 -> Bus Creator/20  "u6"
  Demux/21 -> Bus Creator/21  "u7"
  Demux/22 -> Bus Creator/22  "u8"
  Demux/23 -> Bus Creator/23  "u9"
  Demux/24 -> Bus Creator/24  "u10"
  Demux/25 -> Bus Creator/25  "u11"
  Demux/26 -> Bus Creator/26  "u12"

== system ICW_a1/Veh_1/ComplexVehicleModel/Steer/SteerToBody ==
  In1 : Inport
  Bus Creator : BusCreator  Inputs=7
  Demux : Demux  Outputs=[2 4 4 4 4 4 4]
  Out1 : Outport
  wires:
  In1/1 -> Demux/1
  Demux/1 -> Bus Creator/1  "strratio"
  Demux/2 -> Bus Creator/2  "strc_str"
  Demux/3 -> Bus Creator/3  "kppc_str"
  Demux/4 -> Bus Creator/4  "kprc_str"
  Demux/5 -> Bus Creator/5  "rotd_kp_dr_str"
  Demux/6 -> Bus Creator/6  "rotd_kp_susp_str"
  Demux/7 -> Bus Creator/7  "gear_rotd_susp_str"
  Bus Creator/1 -> Out1/1  "Steer2Body"

== system ICW_a1/Veh_1/ComplexVehicleModel/Suspensions/SupensionsStates ==
  In1 : Inport
  Bus Creator : BusCreator  Inputs=32
  Demux : Demux  Outputs=32
  Out1 : Outport
  wires:
  In1/1 -> Demux/1
  Demux/1 -> Bus Creator/1  "q0"
  Demux/2 -> Bus Creator/2  "q1"
  Demux/3 -> Bus Creator/3  "q2"
  Demux/4 -> Bus Creator/4  "q3"
  Demux/5 -> Bus Creator/5  "q4"
  Demux/6 -> Bus Creator/6  "q5"
  Demux/7 -> Bus Creator/7  "q6"
  Demux/8 -> Bus Creator/8  "q7"
  Demux/9 -> Bus Creator/9  "q8"
  Demux/10 -> Bus Creator/10  "q9"
  Demux/11 -> Bus Creator/11  "q10"
  Demux/12 -> Bus Creator/12  "q11"
  Demux/13 -> Bus Creator/13  "q12"
  Demux/14 -> Bus Creator/14  "q13"
  Demux/15 -> Bus Creator/15  "q14"
  Demux/16 -> Bus Creator/16  "q15"
  Bus Creator/1 -> Out1/1  "Suspensions States"
  Demux/17 -> Bus Creator/17  "u0"
  Demux/18 -> Bus Creator/18  "u1"
  Demux/19 -> Bus Creator/19  "u2"
  Demux/20 -> Bus Creator/20  "u3"
  Demux/21 -> Bus Creator/21  "u4"
  Demux/22 -> Bus Creator/22  "u5"
  Demux/23 -> Bus Creator/23  "u6"
  Demux/24 -> Bus Creator/24  "u7"
  Demux/25 -> Bus Creator/25  "u8"
  Demux/26 -> Bus Creator/26  "u9"
  Demux/27 -> Bus Creator/27  "u10"
  Demux/28 -> Bus Creator/28  "u11"
  Demux/29 -> Bus Creator/29  "u12"
  Demux/30 -> Bus Creator/30  "u13"
  Demux/31 -> Bus Creator/31  "u14"
  Demux/32 -> Bus Creator/32  "u15"

== system ICW_a1/Veh_1/ComplexVehicleModel/Suspensions/SuspensionForces ==
  In1 : Inport
  Bus Creator : BusCreator  Inputs=18
  Demux : Demux  Outputs=18
  Out1 : Outport
  wires:
  Bus Creator/1 -> Out1/1  "SuspensionForces"
  In1/1 -> Demux/1
  Demux/1 -> Bus Creator/1  "spring_f_r1"
  Demux/2 -> Bus Creator/2  "spring_f_l1"
  Demux/3 -> Bus Creator/3  "spring_f_r2"
  Demux/4 -> Bus Creator/4  "spring_f_l2"
  Demux/5 -> Bus Creator/5  "jounce_stop_f_r1"
  Demux/6 -> Bus Creator/6  "reound_stop_f_r1"
  Demux/7 -> Bus Creator/7  "jounce_stop_f_l1"
  Demux/8 -> Bus Creator/8  "reound_stop_f_l1"
  Demux/9 -> Bus Creator/9  "jounce_stop_f_r2"
  Demux/10 -> Bus Creator/10  "reound_stop_f_r2"
  Demux/11 -> Bus Creator/11  "jounce_stop_f_l2"
  Demux/12 -> Bus Creator/12  "reound_stop_f_l2"
  Demux/13 -> Bus Creator/13  "damper_l1"
  Demux/14 -> Bus Creator/14  "damper_r1"
  Demux/15 -> Bus Creator/15  "damper_l2"
  Demux/16 -> Bus Creator/16  "damper_r2"
  Demux/17 -> Bus Creator/17  "maux_f"
  Demux/18 -> Bus Creator/18  "maux_r"

== system ICW_a1/Veh_1/ComplexVehicleModel/Suspensions/SuspensionKinematics ==
  In1 : Inport
  Bus Creator : BusCreator  Inputs=23
  Demux : Demux  Outputs=[4 4 4 4 4 4 4 4 4 4 4 4 4 4 4 4 4 4 4 4 4 4 4]
  Out1 : Outport
  wires:
  Demux/23 -> Bus Creator/23  "fs_ext_susp"
  Demux/22 -> Bus Creator/22  "fs_susp"
  Demux/21 -> Bus Creator/21  "cmp_s_susp"
  Demux/20 -> Bus Creator/20  "cmprst_susp"
  Demux/19 -> Bus Creator/19  "cmprd_susp"
  Demux/18 -> Bus Creator/18  "cmpjst_susp"
  Demux/17 -> Bus Creator/17  "dcam_con_susp"
  Bus Creator/1 -> Out1/1  "SuspensionsKinematiocs"
  Demux/16 -> Bus Creator/16  "divedd_susp"
  Demux/15 -> Bus Creator/15  "dived_susp"
  Demux/14 -> Bus Creator/14  "dive_susp"
  Demux/13 -> Bus Creator/13  "toedd_susp"
  Demux/12 -> Bus Creator/12  "toed_susp"
  Demux/11 -> Bus Creator/11  "toe_susp"
  Demux/10 -> Bus Creator/10  "camdd_susp"
  Demux/9 -> Bus Creator/9  "camd_susp"
  Demux/8 -> Bus Creator/8  "cam_con_susp"
  Demux/7 -> Bus Creator/7  "cam_susp"
  Demux/6 -> Bus Creator/6  "latdd_susp"
  Demux/5 -> Bus Creator/5  "latd_susp"
  Demux/4 -> Bus Creator/4  "lat_susp"
  Demux/3 -> Bus Creator/3  "xdd_susp"
  Demux/2 -> Bus Creator/2  "xd_susp"
  Demux/1 -> Bus Creator/1  "x_susp"
  In1/1 -> Demux/1

== system ICW_a1/Veh_1/ComplexVehicleModel/Suspensions/SuspensionSteer ==
  In1 : Inport
  Bus Creator : BusCreator  Inputs=3
  Demux : Demux  Outputs=[4 4 4]
  Out1 : Outport
  wires:
  Bus Creator/1 -> Out1/1  "SuspensionSteer"
  Demux/3 -> Bus Creator/3  "sw_mz_susp"
  Demux/2 -> Bus Creator/2  "sw_fy_susp"
  Demux/1 -> Bus Creator/1  "sw_fx_susp"
  In1/1 -> Demux/1

== system ICW_a1/Veh_1/DriverModel/Driver/Driver2Brake ==
  In1 : Inport
  Bus Creator : BusCreator  Inputs=1
  Demux : Demux  Outputs=1
  Out1 : Outport
  wires:
  In1/1 -> Demux/1
  Demux/1 -> Bus Creator/1  "pcon_bk"
  Bus Creator/1 -> Out1/1  "Driver2Brake"

== system ICW_a1/Veh_1/DriverModel/Driver/Driver2Powertrain ==
  In1 : Inport
  Bus Creator : BusCreator  Inputs=3
  Demux : Demux  Outputs=3
  Out1 : Outport
  wires:
  Bus Creator/1 -> Out1/1  "Driver2Powertrain"
  Demux/1 -> Bus Creator/1  "throttle"
  In1/1 -> Demux/1
  Demux/2 -> Bus Creator/2  "modetr"
  Demux/3 -> Bus Creator/3  "geartr"

== system ICW_a1/Veh_1/DriverModel/Driver/Driver2Steer ==
  In1 : Inport
  Bus Creator : BusCreator  Inputs=1
  Demux : Demux  Outputs=1
  Out1 : Outport
  wires:
  In1/1 -> Demux/1
  Demux/1 -> Bus Creator/1  "drstr_drv"
  Bus Creator/1 -> Out1/1  "Driver2Steer"

== system ICW_a1/Veh_1/DriverModel/Driver/DriverStates ==
  In1 : Inport
  Bus Creator : BusCreator  Inputs=4
  Demux : Demux
  Out1 : Outport
  wires:
  Bus Creator/1 -> Out1/1  "DriverStates"
  Demux/4 -> Bus Creator/4  "my_sc_r"
  Demux/3 -> Bus Creator/3  "my_sc_f"
  Demux/2 -> Bus Creator/2  "verr_drv"
  Demux/1 -> Bus Creator/1  "iverr_drv"
  In1/1 -> Demux/1

== system ICW_a1/Veh_1_1/ComplexVehicleModel/Aerodynamics/Chassis States ==
  In1 : Inport
  Bus Creator : BusCreator  Inputs=12
  Demux : Demux  Outputs=12
  Out1 : Outport
  wires:
  In1/1 -> Demux/1
  Demux/1 -> Bus Creator/1  "beta_air"
  Demux/2 -> Bus Creator/2  "pitch_air"
  Demux/3 -> Bus Creator/3  "yawwind_air"
  Demux/4 -> Bus Creator/4  "v_air"
  Demux/5 -> Bus Creator/5  "vwind_air"
  Demux/6 -> Bus Creator/6  "z_air"
  Demux/7 -> Bus Creator/7  "fx_air"
  Demux/8 -> Bus Creator/8  "fy_air"
  Demux/9 -> Bus Creator/9  "fz_air"
  Demux/10 -> Bus Creator/10  "mx_air"
  Demux/11 -> Bus Creator/11  "my_air"
  Demux/12 -> Bus Creator/12  "mz_air"
  Bus Creator/1 -> Out1/1  "Aerodynamics_States"

== system ICW_a1/Veh_1_1/ComplexVehicleModel/Body and Tires/Body ==
  Aero Input : Inport
  Susp Input : Inport  Port=2
  Steer Input : Inport  Port=3
  Power Input : Inport  Port=4
  Brake Input : Inport  Port=5
  Tires Input : Inport  Port=6
  Direct Input : Inport  Port=7
  Body Model : S-Function  FunctionName=panoBody_sfun  Parameters='b7d0cac6-2e70-43e3-a322-7c7b3e2b0354'  SFunctionDeploymentMode=off  EnableBusSupport=off
  Chassis Motion : Subsystem
  Chassis States : Subsystem
  Wheel 1 : Subsystem
  Wheel 2 : Subsystem
  Wheel 3 : Subsystem
  Wheel 4 : Subsystem
  State : Outport
  Chassis : Outport  Port=2
  Wheel LF : Outport  Port=3
  Wheel RF : Outport  Port=4
  Wheel LR : Outport  Port=5
  Wheel RR : Outport  Port=6
  wires:
  Direct Input/1 -> Body Model/7
  Body Model/2 -> Chassis Motion/1(In1)
  Chassis Motion/1(Out1) -> Chassis/1  "Chassis_Motion"
  Body Model/1 -> Chassis States/1(In1)
  Chassis States/1(Out1) -> State/1  "Chassis_States"
  Body Model/3 -> Wheel 1/1(In1)
  Wheel 1/1(Out1) -> Wheel LF/1  "Wheel_LF"
  Body Model/4 -> Wheel 2/1(In1)
  Body Model/5 -> Wheel 3/1(In1)
  Body Model/6 -> Wheel 4/1(In1)
  Wheel 3/1(Out1) -> Wheel LR/1  "Wheel_LR"
  Wheel 4/1(Out1) -> Wheel RR/1  "Wheel_RR"
  Wheel 2/1(Out1) -> Wheel RF/1  "Wheel_RF"
  Tires Input/1 -> Body Model/6
  Power Input/1 -> Body Model/4
  Brake Input/1 -> Body Model/5
  Steer Input/1 -> Body Model/3
  Susp Input/1 -> Body Model/2
  Aero Input/1 -> Body Model/1

== system ICW_a1/Veh_1_1/ComplexVehicleModel/Body and Tires/Tires ==
  Wheel LF : Inport
  Wheel RF : Inport  Port=2
  Wheel LR : Inport  Port=3
  Wheel RR : Inport  Port=4
  Tires Force  2 : Subsystem
  "Tires Force 1 " : Subsystem
  Tires Force 3 : Subsystem
  Tires Force 4 : Subsystem
  Tires Force Ground : Subsystem
  Tires Model : S-Function  FunctionName=panoTire_sfun  Parameters='b7d0cac6-2e70-43e3-a322-7c7b3e2b0354'  SFunctionDeploymentMode=off  EnableBusSupport=off
  TiresStates : Subsystem
  Tire States : Outport
  Tire LF : Outport  Port=2
  Tire RF : Outport  Port=3
  Tire LR : Outport  Port=4
  Tire RR : Outport  Port=5
  Tire Force Ground : Outport  Port=6
  wires:
  Tires Model/6 -> Tires Force Ground/1(In1)
  Tires Force Ground/1(Out1) -> Tire Force Ground/1  "Tire_Forces_GND"
  Wheel LF/1 -> Tires Model/1
  Wheel RF/1 -> Tires Model/2
  Wheel LR/1 -> Tires Model/3
  Wheel RR/1 -> Tires Model/4
  Tires Model/1 -> TiresStates/1(In1)
  TiresStates/1(Out1) -> Tire States/1  "Tires_States"
  Tires Model/2 -> "Tires Force 1 "/1(In1)
  "Tires Force 1 "/1(Out1) -> Tire LF/1  "Tire_Forces_LF"
  Tires Model/5 -> Tires Force 4/1(In1)
  Tires Model/4 -> Tires Force 3/1(In1)
  Tires Model/3 -> Tires Force  2/1(In1)
  Tires Force 3/1(Out1) -> Tire LR/1  "Tire_Forces_LR"
  Tires Force 4/1(Out1) -> Tire RR/1  "Tire_Forces_RR"
  Tires Force  2/1(Out1) -> Tire RF/1  "Tire_Forces_RF"

== system ICW_a1/Veh_1_1/ComplexVehicleModel/Body and Tires/body_kinematic_out_whl_lf ==
  In1 : Inport
  Bus Creator : BusCreator  Inputs=18
  Demux : Demux  Outputs=18
  Out1 : Outport
  wires:
  In1/1 -> Demux/1
  Demux/1 -> Bus Creator/1  "rot_whl"
  Demux/2 -> Bus Creator/2  "w_whl"
  Demux/3 -> Bus Creator/3  "z_whl_whl"
  Demux/4 -> Bus Creator/4  "yaw_whl"
  Demux/5 -> Bus Creator/5  "pitch_whl"
  Demux/6 -> Bus Creator/6  "roll_whl"
  Demux/7 -> Bus Creator/7  "vwx_whl"
  Demux/8 -> Bus Creator/8  "vwy_whl"
  Demux/9 -> Bus Creator/9  "vwz_whl"
  Demux/10 -> Bus Creator/10  "avwx_whl"
  Demux/11 -> Bus Creator/11  "avwy_whl"
  Demux/12 -> Bus Creator/12  "avwz_whl"
  Demux/13 -> Bus Creator/13  "dzdx_whl"
  Demux/14 -> Bus Creator/14  "dzdy_whl"
  Demux/15 -> Bus Creator/15  "xgnd_whl"
  Demux/16 -> Bus Creator/16  "ygnd_whl"
  Demux/17 -> Bus Creator/17  "zgnd_whl"
  Demux/18 -> Bus Creator/18  "mux_whl"
  Bus Creator/1 -> Out1/1  "bodykin_whl_out"

== system ICW_a1/Veh_1_1/ComplexVehicleModel/Body and Tires/body_kinematic_out_whl_lf1 ==
  In1 : Inport
  Bus Creator : BusCreator  Inputs=18
  Demux : Demux  Outputs=18
  Out1 : Outport
  wires:
  Bus Creator/1 -> Out1/1  "bodykin_whl_out"
  Demux/18 -> Bus Creator/18  "mux_whl"
  Demux/17 -> Bus Creator/17  "zgnd_whl"
  Demux/16 -> Bus Creator/16  "ygnd_whl"
  Demux/15 -> Bus Creator/15  "xgnd_whl"
  Demux/14 -> Bus Creator/14  "dzdy_whl"
  Demux/13 -> Bus Creator/13  "dzdx_whl"
  Demux/12 -> Bus Creator/12  "avwz_whl"
  Demux/11 -> Bus Creator/11  "avwy_whl"
  Demux/10 -> Bus Creator/10  "avwx_whl"
  Demux/9 -> Bus Creator/9  "vwz_whl"
  Demux/8 -> Bus Creator/8  "vwy_whl"
  Demux/7 -> Bus Creator/7  "vwx_whl"
  Demux/6 -> Bus Creator/6  "roll_whl"
  Demux/5 -> Bus Creator/5  "pitch_whl"
  Demux/4 -> Bus Creator/4  "yaw_whl"
  Demux/3 -> Bus Creator/3  "z_whl_whl"
  Demux/2 -> Bus Creator/2  "w_whl"
  Demux/1 -> Bus Creator/1  "rot_whl"
  In1/1 -> Demux/1

== system ICW_a1/Veh_1_1/ComplexVehicleModel/Body and Tires/body_kinematic_out_whl_lf2 ==
  In1 : Inport
  Bus Creator : BusCreator  Inputs=18
  Demux : Demux  Outputs=18
  Out1 : Outport
  wires:
  In1/1 -> Demux/1
  Demux/1 -> Bus Creator/1  "rot_whl"
  Demux/2 -> Bus Creator/2  "w_whl"
  Demux/3 -> Bus Creator/3  "z_whl_whl"
  Demux/4 -> Bus Creator/4  "yaw_whl"
  Demux/5 -> Bus Creator/5  "pitch_whl"
  Demux/6 -> Bus Creator/6  "roll_whl"
  Demux/7 -> Bus Creator/7  "vwx_whl"
  Demux/8 -> Bus Creator/8  "vwy_whl"
  Demux/9 -> Bus Creator/9  "vwz_whl"
  Demux/10 -> Bus Creator/10  "avwx_whl"
  Demux/11 -> Bus Creator/11  "avwy_whl"
  Demux/12 -> Bus Creator/12  "avwz_whl"
  Demux/13 -> Bus Creator/13  "dzdx_whl"
  Demux/14 -> Bus Creator/14  "dzdy_whl"
  Demux/15 -> Bus Creator/15  "xgnd_whl"
  Demux/16 -> Bus Creator/16  "ygnd_whl"
  Demux/17 -> Bus Creator/17  "zgnd_whl"
  Demux/18 -> Bus Creator/18  "mux_whl"
  Bus Creator/1 -> Out1/1  "bodykin_whl_out"

== system ICW_a1/Veh_1_1/ComplexVehicleModel/Body and Tires/body_kinematic_out_whl_lf3 ==
  In1 : Inport
  Bus Creator : BusCreator  Inputs=18
  Demux : Demux  Outputs=18
  Out1 : Outport
  wires:
  Bus Creator/1 -> Out1/1  "bodykin_whl_out"
  Demux/18 -> Bus Creator/18  "mux_whl"
  Demux/17 -> Bus Creator/17  "zgnd_whl"
  Demux/16 -> Bus Creator/16  "ygnd_whl"
  Demux/15 -> Bus Creator/15  "xgnd_whl"
  Demux/14 -> Bus Creator/14  "dzdy_whl"
  Demux/13 -> Bus Creator/13  "dzdx_whl"
  Demux/12 -> Bus Creator/12  "avwz_whl"
  Demux/11 -> Bus Creator/11  "avwy_whl"
  Demux/10 -> Bus Creator/10  "avwx_whl"
  Demux/9 -> Bus Creator/9  "vwz_whl"
  Demux/8 -> Bus Creator/8  "vwy_whl"
  Demux/7 -> Bus Creator/7  "vwx_whl"
  Demux/6 -> Bus Creator/6  "roll_whl"
  Demux/5 -> Bus Creator/5  "pitch_whl"
  Demux/4 -> Bus Creator/4  "yaw_whl"
  Demux/3 -> Bus Creator/3  "z_whl_whl"
  Demux/2 -> Bus Creator/2  "w_whl"
  Demux/1 -> Bus Creator/1  "rot_whl"
  In1/1 -> Demux/1

== system ICW_a1/Veh_1_1/ComplexVehicleModel/Brake/Brake States ==
  In1 : Inport
  Bus Creator : BusCreator  Inputs=26
  Demux : Demux  Outputs=26
  Out1 : Outport
  wires:
  In1/1 -> Demux/1
  Demux/1 -> Bus Creator/1  "q0"
  Demux/2 -> Bus Creator/2  "q1"
  Demux/3 -> Bus Creator/3  "q2"
  Demux/4 -> Bus Creator/4  "q3"
  Demux/5 -> Bus Creator/5  "q4"
  Demux/6 -> Bus Creator/6  "q5"
  Demux/7 -> Bus Creator/7  "q6"
  Demux/8 -> Bus Creator/8  "q7"
  Demux/9 -> Bus Creator/9  "q8"
  Demux/10 -> Bus Creator/10  "q9"
  Demux/11 -> Bus Creator/11  "q10"
  Demux/12 -> Bus Creator/12  "q11"
  Demux/13 -> Bus Creator/13  "q12"
  Demux/14 -> Bus Creator/14  "u0"
  Demux/15 -> Bus Creator/15  "u1"
  Demux/16 -> Bus Creator/16  "u2"
  Bus Creator/1 -> Out1/1  "BrakeStates"
  Demux/17 -> Bus Creator/17  "u3"
  Demux/18 -> Bus Creator/18  "u4"
  Demux/19 -> Bus Creator/19  "u5"
  Demux/20 -> Bus Creator/20  "u6"
  Demux/21 -> Bus Creator/21  "u7"
  Demux/22 -> Bus Creator/22  "u8"
  Demux/23 -> Bus Creator/23  "u9"
  Demux/24 -> Bus Creator/24  "u10"
  Demux/25 -> Bus Creator/25  "u11"
  Demux/26 -> Bus Creator/26  "u12"

== system ICW_a1/Veh_1_1/ComplexVehicleModel/Brake/SteerStates1 ==
  In1 : Inport
  Bus Creator : BusCreator  Inputs=22
  Demux : Demux  Outputs=22
  Out1 : Outport
  wires:
  Demux/22 -> Bus Creator/22  "turn_off"
  Demux/21 -> Bus Creator/21  "brake"
  Demux/20 -> Bus Creator/20  "trot_brk_rr"
  Demux/19 -> Bus Creator/19  "trot_brk_lr"
  Demux/18 -> Bus Creator/18  "trot_brk_rf"
  Demux/17 -> Bus Creator/17  "trot_brk_lf"
  Bus Creator/1 -> Out1/1  "BrakeOutput"
  Demux/16 -> Bus Creator/16  "mu_us_brk_rr"
  Demux/15 -> Bus Creator/15  "mu_us_brk_lr"
  Demux/14 -> Bus Creator/14  "mu_us_brk_rf"
  Demux/13 -> Bus Creator/13  "mu_us_brk_lf"
  Demux/12 -> Bus Creator/12  "fm_brk_rr"
  Demux/11 -> Bus Creator/11  "fm_brk_lr"
  Demux/10 -> Bus Creator/10  "fm_brk_rf"
  Demux/9 -> Bus Creator/9  "fm_brk_lf"
  Demux/8 -> Bus Creator/8  "pbkch_brk_rr"
  Demux/7 -> Bus Creator/7  "pbkch_brk_lr"
  Demux/6 -> Bus Creator/6  "pbkch_brk_rf"
  Demux/5 -> Bus Creator/5  "pbkch_brk_lf"
  Demux/4 -> Bus Creator/4  "fbk_out_brk"
  Demux/3 -> Bus Creator/3  "fbk_in_brk"
  Demux/2 -> Bus Creator/2  "fbk_pedal"
  Demux/1 -> Bus Creator/1  "pbk_con_brk"
  In1/1 -> Demux/1

== system ICW_a1/Veh_1_1/ComplexVehicleModel/Powertrain/PowertrainOut ==
  In1 : Inport
  Bus Creator : BusCreator  Inputs=36
  Demux : Demux  Outputs=36
  Out1 : Outport
  wires:
  Bus Creator/1 -> Out1/1  "PowertrainOut"
  In1/1 -> Demux/1
  Demux/1 -> Bus Creator/1  "aa_eng"
  Demux/2 -> Bus Creator/2  "av_eng"
  Demux/3 -> Bus Creator/3  "av_eng_update"
  Demux/4 -> Bus Creator/4  "av_tc"
  Demux/5 -> Bus Creator/5  "fuel"
  Demux/6 -> Bus Creator/6  "iw_eff_pt_lf"
  Demux/7 -> Bus Creator/7  "iw_eff_pt_rf"
  Demux/8 -> Bus Creator/8  "iw_eff_pt_lr"
  Demux/9 -> Bus Creator/9  "iw_eff_pt_rr"
  Demux/10 -> Bus Creator/10  "my_drv_lf"
  Demux/11 -> Bus Creator/11  "my_drv_rf"
  Demux/12 -> Bus Creator/12  "my_drv_lr"
  Demux/13 -> Bus Creator/13  "my_drv_rr"
  Demux/14 -> Bus Creator/14  "pt_thr_eng"
  Demux/15 -> Bus Creator/15  "pt_throttle"
  Demux/16 -> Bus Creator/16  "pt_modetran"
  Demux/17 -> Bus Creator/17  "pt_rottrans"
  Demux/18 -> Bus Creator/18  "pt_m_engout"
  Demux/19 -> Bus Creator/19  "pt_m_eng_in"
  Demux/20 -> Bus Creator/20  "pt_gearauto"
  Demux/21 -> Bus Creator/21  "pt_gear_status"
  Demux/22 -> Bus Creator/22  "pt_gear_man"
  Demux/23 -> Bus Creator/23  "rot_eng_update"
  Demux/24 -> Bus Creator/24  "rot_tc"
  Demux/25 -> Bus Creator/25  "pt_av_trans"
  Demux/26 -> Bus Creator/26  "pt_m_tc"
  Demux/27 -> Bus Creator/27  "pt_m_trans"
  Demux/28 -> Bus Creator/28  "pt_pwrengin"
  Demux/29 -> Bus Creator/29  "pt_pwrengo"
  Demux/30 -> Bus Creator/30  "pt_pwrtrans"
  Demux/31 -> Bus Creator/31  "pt_pwrwheel"
  Demux/32 -> Bus Creator/32  "pt_pwr_tc"
  Demux/33 -> Bus Creator/33  "pt_clutch"
  Demux/34 -> Bus Creator/34  "pt_k_tc"
  Demux/35 -> Bus Creator/35  "pt_r_av_tc"
  Demux/36 -> Bus Creator/36  "pt_r_m_tc"

== system ICW_a1/Veh_1_1/ComplexVehicleModel/Powertrain/PowertrainStates ==
  In1 : Inport
  Bus Creator : BusCreator  Inputs=38
  Demux : Demux  Outputs=38
  Out1 : Outport
  wires:
  In1/1 -> Demux/1
  Bus Creator/1 -> Out1/1  "PowertrainStates"
  Demux/1 -> Bus Creator/1  "q0"
  Demux/2 -> Bus Creator/2  "q1"
  Demux/3 -> Bus Creator/3  "q2"
  Demux/4 -> Bus Creator/4  "q3"
  Demux/5 -> Bus Creator/5  "q4"
  Demux/6 -> Bus Creator/6  "q5"
  Demux/7 -> Bus Creator/7  "q6"
  Demux/8 -> Bus Creator/8  "q7"
  Demux/9 -> Bus Creator/9  "q8"
  Demux/10 -> Bus Creator/10  "q9"
  Demux/11 -> Bus Creator/11  "q10"
  Demux/12 -> Bus Creator/12  "q11"
  Demux/13 -> Bus Creator/13  "q12"
  Demux/14 -> Bus Creator/14  "q13"
  Demux/15 -> Bus Creator/15  "q14"
  Demux/16 -> Bus Creator/16  "q15"
  Demux/17 -> Bus Creator/17  "q16"
  Demux/18 -> Bus Creator/18  "q17"
  Demux/19 -> Bus Creator/19  "q18"
  Demux/20 -> Bus Creator/20  "u0"
  Demux/21 -> Bus Creator/21  "u1"
  Demux/22 -> Bus Creator/22  "u2"
  Demux/23 -> Bus Creator/23  "u3"
  Demux/24 -> Bus Creator/24  "u4"
  Demux/25 -> Bus Creator/25  "u5"
  Demux/26 -> Bus Creator/26  "u6"
  Demux/27 -> Bus Creator/27  "u7"
  Demux/28 -> Bus Creator/28  "u8"
  Demux/29 -> Bus Creator/29  "u9"
  Demux/30 -> Bus Creator/30  "u10"
  Demux/31 -> Bus Creator/31  "u11"
  Demux/32 -> Bus Creator/32  "u12"
  Demux/33 -> Bus Creator/33  "u13"
  Demux/34 -> Bus Creator/34  "u14"
  Demux/35 -> Bus Creator/35  "u15"
  Demux/36 -> Bus Creator/36  "u16"
  Demux/37 -> Bus Creator/37  "u17"
  Demux/38 -> Bus Creator/38  "u18"
